simulink model "ControlRobot"  (R2018a)
settings: Solver=FixedStepAuto  StartTime=0.0  StopTime=3  FixedStep=T  RelTol=1e-3
values from neighbouring files (symbols this model uses):
  Bv = 0.055    [F.m]    (also in FNew.m = 0.038709; Project.m = 0.55; ProjectEdit.m = 0.55; SimulationWorkspace.m = 0.038709)
  Bvc = 0.038709    [SimulationWorkspace.m]
  Bw = 0.015    [F.m]    (also in FNew.m = 0.0008517; Project.m; ProjectEdit.m; SimulationWorkspace.m = 0.0008517)
  Bwc = 0.0008517    [SimulationWorkspace.m]
  Cv = 0.2    [F.m]    (also in FNew.m = 0.019178; Project.m = 2; ProjectEdit.m = 2; SimulationWorkspace.m = 0.019178)
  Cvc = 0.019178    [SimulationWorkspace.m]
  Cw = 0.14    [F.m]    (also in FNew.m = 0.099875; Project.m; ProjectEdit.m; SimulationWorkspace.m = 0.099875)
  Cwc = 0.099875    [SimulationWorkspace.m]
  eta1 = 1    [SimulationWorkspace.m]
  eta2 = 1    [SimulationWorkspace.m]
  eta3 = 0.1    [SimulationWorkspace.m]
  g = 9.81    [F.m]    (also in FNew.m; ForwardDynamicModel.m; Project.m; ProjectEdit.m)
  j = i + 1    [Fusion.m]
  J = 0.015    [F.m]    (also in FNew.m = 0.002; Jacobian.m = 0.5*[-S, -C, S, C; Project.m; ProjectEdit.m)
  Jc = 0.45923    [SimulationWorkspace.m]
  K1 = 2.5    [SimulationWorkspace.m]
  K2 = 2.5    [SimulationWorkspace.m]
  K3 = 20    [SimulationWorkspace.m]
  L = 0.1    [F.m]    (also in FNew.m = 0.15; H.m = 0.15; Project.m; ProjectEdit.m)
  lambda1 = 2.75    [SimulationWorkspace.m]
  lambda2 = 2.75    [SimulationWorkspace.m]
  lambda3 = 10    [SimulationWorkspace.m]
  M = 6    [F.m]    (also in FNew.m = 9.1; Project.m; ProjectEdit.m; SimulationWorkspace.m = 9.1)
  Mc = 9.1    [SimulationWorkspace.m]
  mu_p = 0    [SimulationWorkspace.m]
  Q = zeros(4, N - 1)    [Project.m]    (also in ProjectEdit.m; SimulationWorkspace.m = diag([0.002, 0.002, 3e-03, 0.002, 0.002, 3e-03]))
  r = 0.05    [F.m]    (also in FNew.m; H.m; Project.m; ProjectEdit.m)
  RG = diag([5e-7, 5e-7, 5e-7])    [SimulationWorkspace.m]
  RH = diag([2.5e-5, 2.5e-5, 2.5e-5, 2.5e-5])    [SimulationWorkspace.m]
  T = [1/29.56, 1/29.43, 1/30, 1/29.43, 1/29.78, 1/29.75, 1/29.8, 1/29.3, 1/29.18, 1/29.74, 1/29.29, 1/29.3, 1/29.73, 1/29.14, 1/29.75]    [DataRead.m]    (also in Encoder.m = 0.02; F.m = u(5); FNew.m = u(5); Fusion.m = 0.01)
libraries: simulink x4, sharedTrackingLibrary x1, dspsrcs4 x1
settings Model: Creator=Ammar Issa  LastModifiedBy=Ammar Issa
settings SolverCC: AlgebraicLoopSolver=LineSearch

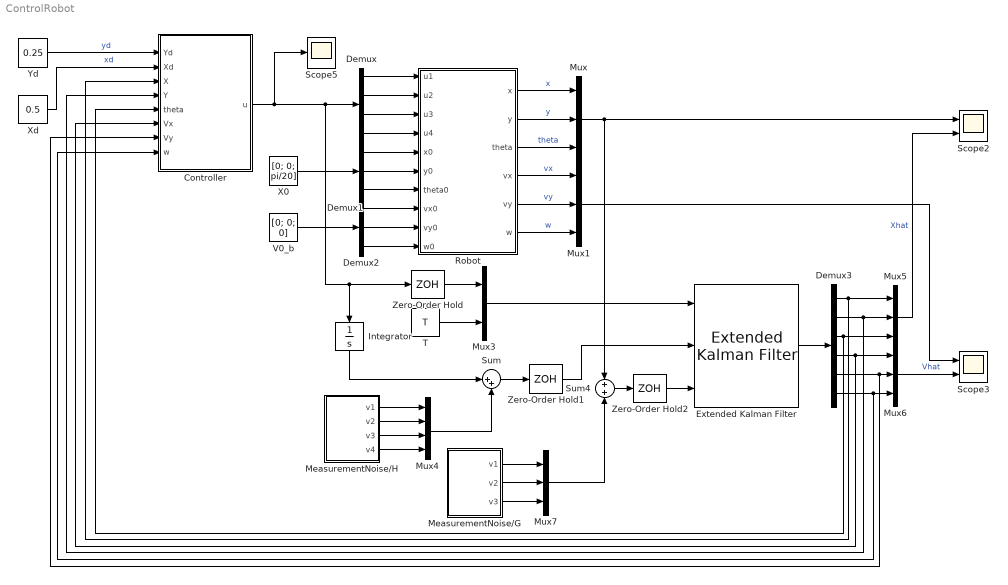
== system ControlRobot ==
  Controller : Subsystem
  Demux : Demux
  Demux1 : Demux  Outputs=3
  Demux2 : Demux  Outputs=3
  Demux3 : Demux  Outputs=6
  Extended Kalman Filter : sharedTrackingLibrary/Extended Kalman Filter  StateTransitionFcn=FNew  HasStateTransitionJacobianFcn=off  HasAdditiveProcessNoise=Additive  ProcessNoise=Q  HasTimeVaryingProcessNoise=off  HasStateTransitionFcnExtraArgument=1  InitialState=[0; 0; pi/20; 0; 0; 0]  InitialStateCovariance=diag([0,0,0,1e-6,1e-6,0])  MeasurementFcn1=H  HasMeasurementJacobianFcn1=off  HasMeasurementEnablePort1=off  HasAdditiveMeasurementNoise1=Additive  MeasurementNoise1=RH  HasTimeVaryingMeasurementNoise1=off  HasMeasurementFcnExtraArgument1=0  MeasurementFcn2=G  HasMeasurementJacobianFcn2=off  HasMeasurementEnablePort2=off  HasAdditiveMeasurementNoise2=Additive  MeasurementNoise2=RG  HasTimeVaryingMeasurementNoise2=off  HasMeasurementFcnExtraArgument2=0  MeasurementFcn3=myMeasurementFcn  HasMeasurementJacobianFcn3=off  HasMeasurementEnablePort3=off  HasAdditiveMeasurementNoise3=Additive  MeasurementNoise3=1  HasTimeVaryingMeasurementNoise3=off  HasMeasurementFcnExtraArgument3=0  MeasurementFcn4=myMeasurementFcn  HasMeasurementJacobianFcn4=off  HasMeasurementEnablePort4=off  HasAdditiveMeasurementNoise4=Additive  MeasurementNoise4=1  HasTimeVaryingMeasurementNoise4=off  HasMeasurementFcnExtraArgument4=0  MeasurementFcn5=myMeasurementFcn  HasMeasurementJacobianFcn5=off  HasMeasurementEnablePort5=off  HasAdditiveMeasurementNoise5=Additive  MeasurementNoise5=1  HasTimeVaryingMeasurementNoise5=off  HasMeasurementFcnExtraArgument5=0  EnableMultirate=on  StateTransitionFcnSampleTime=T  MeasurementFcn1SampleTime=T  MeasurementFcn2SampleTime=T  MeasurementFcn3SampleTime=1  MeasurementFcn4SampleTime=1  MeasurementFcn5SampleTime=1  UseCurrentEstimator=on  OutputStateCovariance=off  DataType=double  SampleTime=T  NumberOfMeasurements=2
      settings: SourceProductName=Control System Toolbox  SourceProductBaseCode=CT
  Integrator : Integrator
  MeasurementNoise/G : Subsystem
  MeasurementNoise/H : Subsystem
  Mux{,1,5..7} (5 alike) : Mux  Inputs=3
  Mux3 : Mux  Inputs=2
  Mux4 : Mux
  Robot : Subsystem
  Scope2 : Scope  NumInputPorts=2
  Scope3 : Scope  NumInputPorts=2
  Scope5 : Scope
  Sum : Sum  Inputs=|++
  Sum4 : Sum
  T : Constant  Value=T
  V0_b : Constant  Value=[0; 0; 0]
  X0 : Constant  Value=[0; 0; pi/20]
  Xd : Constant  Value=0.5
  Yd : Constant  Value=0.25
  Zero-Order Hold : ZeroOrderHold  SampleTime=T
  Zero-Order Hold1 : ZeroOrderHold  SampleTime=T
  Zero-Order Hold2 : ZeroOrderHold  SampleTime=T
  wires:
  Demux1/2 -> Robot/6(y0)
  Sum/1 -> Zero-Order Hold1/1
  Mux5/1 -> Scope2/2  "Xhat"
  T/1 -> Mux3/2
  MeasurementNoise/G/1(v1) -> Mux7/1
  MeasurementNoise/H/1(v1) -> Mux4/1
  Demux3/4 -> Controller/6(Vx), Mux6/1
  MeasurementNoise/H/3(v3) -> Mux4/3
  Mux6/1 -> Scope3/2  "Vhat"
  Mux7/1 -> Sum4/2
  Demux3/3 -> Controller/5(theta), Mux5/3
  Sum4/1 -> Zero-Order Hold2/1
  Demux2/2 -> Robot/9(vy0)
  Zero-Order Hold2/1 -> Extended Kalman Filter/3
  Zero-Order Hold1/1 -> Extended Kalman Filter/2
  Mux/1 -> Scope2/1, Sum4/1
  Zero-Order Hold/1 -> Mux3/1
  Extended Kalman Filter/1 -> Demux3/1
  Demux1/1 -> Robot/5(x0)
  Demux2/3 -> Robot/10(w0)
  Demux/2 -> Robot/2(u2)
  Demux/3 -> Robot/3(u3)
  Robot/4(vx) -> Mux1/1  "vx"
  MeasurementNoise/H/2(v2) -> Mux4/2
  Robot/3(theta) -> Mux/3  "theta"
  MeasurementNoise/H/4(v4) -> Mux4/4
  Robot/1(x) -> Mux/1  "x"
  Demux3/1 -> Controller/3(X), Mux5/1
  V0_b/1 -> Demux2/1
  Mux4/1 -> Sum/2
  Demux2/1 -> Robot/8(vx0)
  X0/1 -> Demux1/1
  MeasurementNoise/G/3(v3) -> Mux7/3
  Demux/1 -> Robot/1(u1)
  Demux3/6 -> Mux6/3, Controller/8(w)
  MeasurementNoise/G/2(v2) -> Mux7/2
  Demux1/3 -> Robot/7(theta0)
  Robot/6(w) -> Mux1/3  "w"
  Mux3/1 -> Extended Kalman Filter/1
  Demux/4 -> Robot/4(u4)
  Mux1/1 -> Scope3/1
  Demux3/5 -> Mux6/2, Controller/7(Vy)
  Robot/2(y) -> Mux/2  "y"
  Demux3/2 -> Controller/4(Y), Mux5/2
  Integrator/1 -> Sum/1
  Robot/5(vy) -> Mux1/2  "vy"
  Controller/1(u) -> Scope5/1, Integrator/1, Zero-Order Hold/1, Demux/1
  Yd/1 -> Controller/1(Yd)  "yd"
  Xd/1 -> Controller/2(Xd)  "xd"

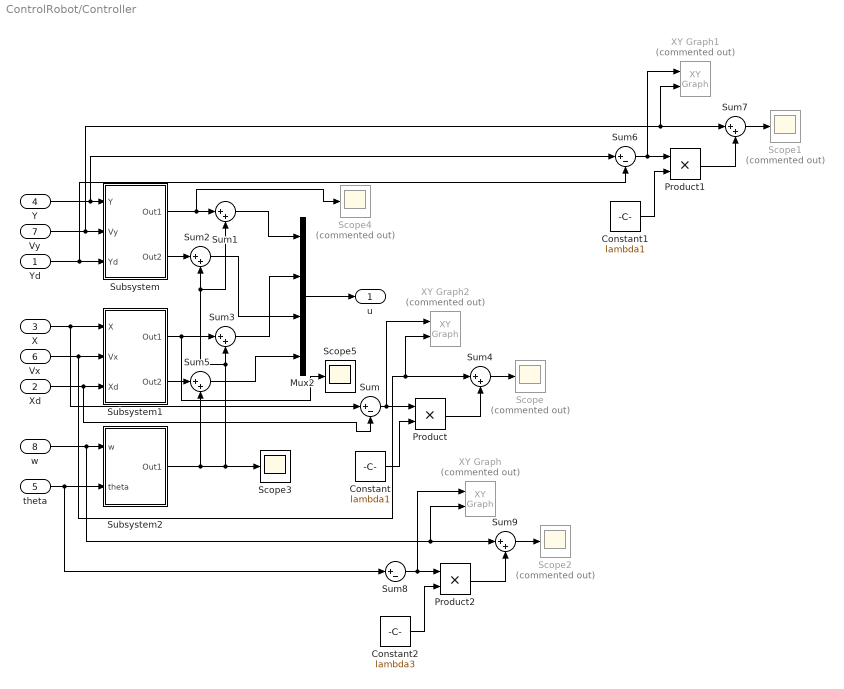
== system ControlRobot/Controller ==
  Yd : Inport
  Xd : Inport  Port=2
  X : Inport  Port=3
  Y : Inport  Port=4
  theta : Inport  Port=5
  Vx : Inport  Port=6
  Vy : Inport  Port=7
  w : Inport  Port=8
  Constant : Constant  Value=lambda1
  Constant1 : Constant  Value=lambda1
  Constant2 : Constant  Value=lambda3
  Mux2 : Mux
  Product : Product
  Product1 : Product
  Product2 : Product
  Scope{,1..2,4} (4 alike) : Scope  Commented=on
  Scope3 : Scope
  Scope5 : Scope
  Subsystem : Subsystem
  Subsystem1 : Subsystem
  Subsystem2 : Subsystem
  Sum : Sum  Inputs=|+-
  Sum{1..5,7,9} (7 alike) : Sum  Inputs=|++
  Sum6 : Sum  Inputs=|+-
  Sum8 : Sum  Inputs=|+-
  XY Graph : simulink/Sinks/XY Graph  Commented=on  xmin=-0.1  xmax=0.2  ymin=-0.05  ymax=0.05  st=-1
  XY Graph1 : simulink/Sinks/XY Graph  Commented=on  xmin=-0.6  xmax=0.1  ymin=-0.1  ymax=1.5  st=-1
  XY Graph2 : simulink/Sinks/XY Graph  Commented=on  xmin=-0.6  xmax=0.1  ymin=-0.1  ymax=1.5  st=-1
  u : Outport
  wires:
  Sum2/1 -> Mux2/3
  Subsystem2/1(Out1) -> Scope3/1, Sum1/2, Sum2/2, Sum3/2, Sum5/2
  Subsystem1/2(Out2) -> Sum5/1
  Subsystem1/1(Out1) -> Scope5/1, Sum3/1
  Subsystem/2(Out2) -> Sum2/1
  Subsystem/1(Out1) -> Scope4/1, Sum1/1
  Sum3/1 -> Mux2/2
  Sum5/1 -> Mux2/4
  Sum1/1 -> Mux2/1
  Xd/1 -> Sum/2, Subsystem1/3(Xd)
  Mux2/1 -> u/1
  Vx/1 -> XY Graph2/2, Sum4/1, Subsystem1/2(Vx)
  X/1 -> Sum/1, Subsystem1/1(X)
  Sum/1 -> XY Graph2/1, Product/1
  Constant/1 -> Product/2
  Product/1 -> Sum4/2
  Sum4/1 -> Scope/1
  Sum7/1 -> Scope1/1
  Product1/1 -> Sum7/2
  Constant1/1 -> Product1/2
  Sum6/1 -> Product1/1, XY Graph1/1
  Y/1 -> Sum6/1, Subsystem/1(Y)
  Vy/1 -> Sum7/1, XY Graph1/2, Subsystem/2(Vy)
  Yd/1 -> Sum6/2, Subsystem/3(Yd)
  Sum9/1 -> Scope2/1
  Product2/1 -> Sum9/2
  Constant2/1 -> Product2/2
  Sum8/1 -> XY Graph/1, Product2/1
  theta/1 -> Sum8/1, Subsystem2/2(theta)
  w/1 -> XY Graph/2, Sum9/1, Subsystem2/1(w)

== system ControlRobot/MeasurementNoise//G ==
  vw1 : RandomNumber  Variance=RG(1, 1)  Seed=4  SampleTime=0
  vw2 : RandomNumber  Variance=RG(2, 2)  Seed=5  SampleTime=0
  vw3 : RandomNumber  Variance=RG(3, 3)  Seed=6  SampleTime=0
  v1 : Outport
  v2 : Outport  Port=2
  v3 : Outport  Port=3
  wires:
  vw1/1 -> v1/1
  vw2/1 -> v2/1
  vw3/1 -> v3/1

== system ControlRobot/MeasurementNoise//H ==
  vw1 : RandomNumber  Variance=RH(1, 1)  SampleTime=0
  vw2 : RandomNumber  Variance=RH(2, 2)  Seed=1  SampleTime=0
  vw3 : RandomNumber  Variance=RH(3, 3)  Seed=2  SampleTime=0
  vw4 : RandomNumber  Variance=RH(4, 4)  Seed=3  SampleTime=0
  v1 : Outport
  v2 : Outport  Port=2
  v3 : Outport  Port=3
  v4 : Outport  Port=4
  wires:
  vw3/1 -> v3/1
  vw4/1 -> v4/1
  vw2/1 -> v2/1
  vw1/1 -> v1/1

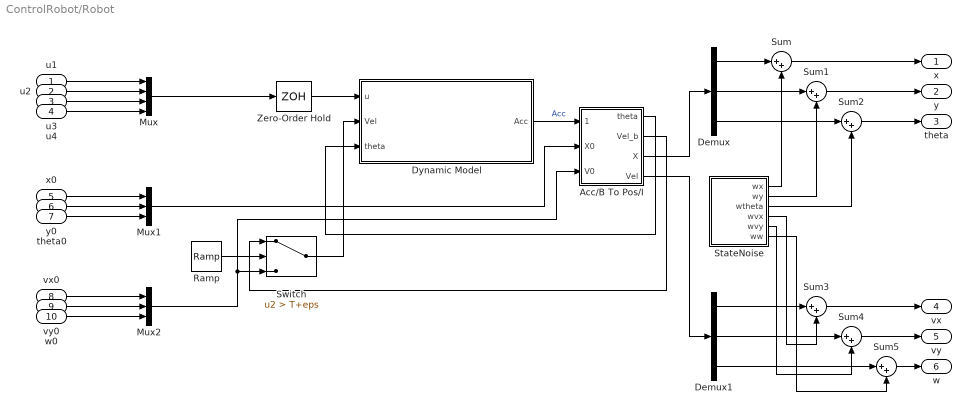
== system ControlRobot/Robot ==
  u1 : Inport
  u2 : Inport  Port=2
  u3 : Inport  Port=3
  u4 : Inport  Port=4
  x0 : Inport  Port=5
  y0 : Inport  Port=6
  theta0 : Inport  Port=7
  vx0 : Inport  Port=8
  vy0 : Inport  Port=9
  w0 : Inport  Port=10
  Acc/B To Pos/I : Subsystem
  Demux : Demux  Outputs=3
  Demux1 : Demux  Outputs=3
  Dynamic Model : Subsystem
  Mux : Mux
  Mux1 : Mux  Inputs=3
  Mux2 : Mux  Inputs=3
  Ramp : simulink/Sources/Ramp  slope=1  start=0  InitialOutput=0
  StateNoise : Subsystem
  Sum{,1..5} (6 alike) : Sum  Inputs=|++
  Switch : Switch  Criteria=u2 > Threshold  Threshold=T+eps
  Zero-Order Hold : ZeroOrderHold  SampleTime=T
  x : Outport
  y : Outport  Port=2
  theta : Outport  Port=3
  vx : Outport  Port=4
  vy : Outport  Port=5
  w : Outport  Port=6
  wires:
  Dynamic Model/1(Acc) -> Acc/B To Pos/I/1(Acc_b)  "Acc"
  Switch/1 -> Dynamic Model/2(Vel)
  Acc/B To Pos/I/1(theta) -> Dynamic Model/3(theta)
  Acc/B To Pos/I/3(X) -> Demux/1
  Mux2/1 -> Acc/B To Pos/I/3(V0), Switch/3
  vx0/1 -> Mux2/1
  Mux1/1 -> Acc/B To Pos/I/2(X0)
  Ramp/1 -> Switch/2
  Acc/B To Pos/I/2(Vel_b) -> Switch/1
  Acc/B To Pos/I/4(Vel) -> Demux1/1
  Mux/1 -> Zero-Order Hold/1
  vy0/1 -> Mux2/2
  u4/1 -> Mux/4
  u3/1 -> Mux/3
  w0/1 -> Mux2/3
  y0/1 -> Mux1/2
  x0/1 -> Mux1/1
  theta0/1 -> Mux1/3
  u2/1 -> Mux/2
  u1/1 -> Mux/1
  Demux/1 -> Sum/1
  Demux/2 -> Sum1/1
  Demux/3 -> Sum2/1
  Demux1/3 -> Sum5/1
  Demux1/2 -> Sum4/1
  Demux1/1 -> Sum3/1
  StateNoise/1(wx) -> Sum/2
  StateNoise/2(wy) -> Sum1/2
  StateNoise/3(wtheta) -> Sum2/2
  StateNoise/4(wvx) -> Sum3/2
  StateNoise/5(wvy) -> Sum4/2
  StateNoise/6(ww) -> Sum5/2
  Sum5/1 -> w/1
  Sum4/1 -> vy/1
  Sum3/1 -> vx/1
  Sum2/1 -> theta/1
  Sum1/1 -> y/1
  Sum/1 -> x/1
  Zero-Order Hold/1 -> Dynamic Model/1(u)

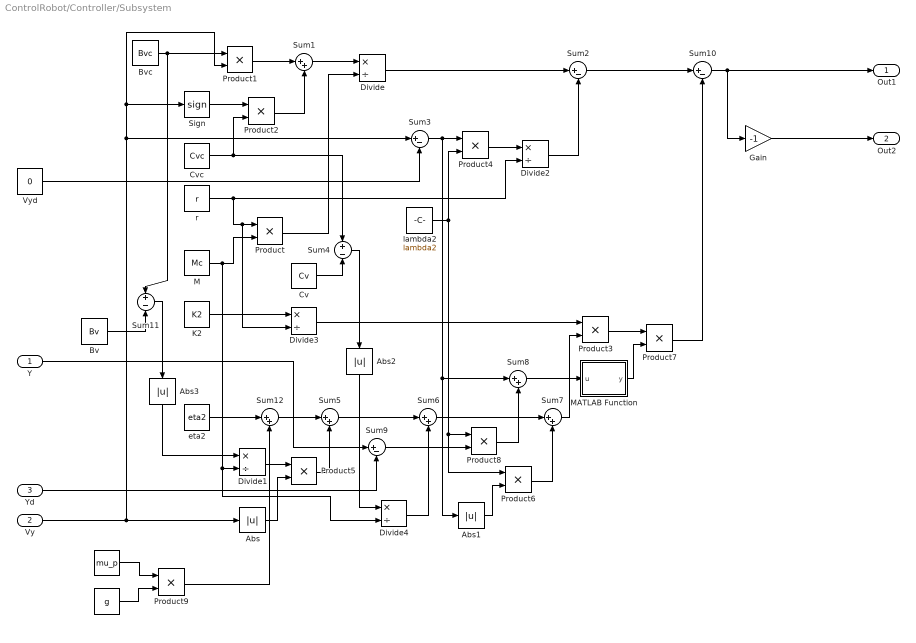
== system ControlRobot/Controller/Subsystem ==
  Y : Inport
  Vy : Inport  Port=2
  Yd : Inport  Port=3
  " " : Constant  Value=mu_p
  "  " : Constant  Value=g
  Abs{,1..3} (4 alike) : Abs
  Bv : Constant  Value=Bv
  Bvc : Constant  Value=Bvc
  Cv : Constant  Value=Cv
  Cvc : Constant  Value=Cvc
  Divide{,1..4} (5 alike) : Product  Inputs=*/
  Gain : Gain  Gain=-1
  K2 : Constant  Value=K2
  M : Constant  Value=Mc
  MATLAB Function : MATLAB Function  TreatAsAtomicUnit=on
  Product{,1..9} (10 alike) : Product
  Sign : Signum
  Sum{1,5..8,12} (6 alike) : Sum  Inputs=|++
  Sum{2..3,9..10} (4 alike) : Sum  Inputs=|+-
  Sum11 : Sum  Inputs=+-
  Sum4 : Sum  Inputs=+-
  Vyd : Constant  Value=0
  eta2 : Constant  Value=eta2
  lambda2 : Constant  Value=lambda2
  r : Constant  Value=r
  Out1 : Outport
  Out2 : Outport  Port=2
  wires:
  Divide4/1 -> Sum6/2
  Product4/1 -> Divide2/1
  Bvc/1 -> Sum11/1, Product1/1
  Divide/1 -> Sum2/1
  Sum1/1 -> Divide/1
  Vy/1 -> Sign/1, Product1/2, Sum3/1, Abs/1
  Sum5/1 -> Sum6/1
  Product3/1 -> Product7/1
  Abs1/1 -> Product6/2
  Product8/1 -> Sum8/2
  Sum9/1 -> Product8/2
  Sum3/1 -> Sum8/1, Abs1/1, Product4/1
  Abs/1 -> Product5/2
  Sum7/1 -> Product3/2
  lambda2/1 -> Product8/1, Product6/1, Product4/2
  Product7/1 -> Sum10/2
  Y/1 -> Sum9/1
  Product1/1 -> Sum1/1
  MATLAB Function/1(y) -> Product7/2
  Sum6/1 -> Sum7/1
  Sum2/1 -> Sum10/1
  M/1 -> Divide1/2, Divide4/2, Product/2
  Product6/1 -> Sum7/2
  Sign/1 -> Product2/1
  Sum10/1 -> Out1/1, Gain/1
  r/1 -> Divide2/2, Divide3/2, Product/1
  Product2/1 -> Sum1/2
  Divide1/1 -> Product5/1
  Product5/1 -> Sum5/2
  Product/1 -> Divide/2
  Divide2/1 -> Sum2/2
  Cvc/1 -> Sum4/1, Product2/2
  K2/1 -> Divide3/1
  Divide3/1 -> Product3/1
  Yd/1 -> Sum9/2
  Gain/1 -> Out2/1
  Vyd/1 -> Sum3/2
  Sum8/1 -> MATLAB Function/1(u)
  Cv/1 -> Sum4/2
  Sum4/1 -> Abs2/1
  Abs2/1 -> Divide4/1
  Bv/1 -> Sum11/2
  Sum11/1 -> Abs3/1
  Abs3/1 -> Divide1/1
  eta2/1 -> Sum12/1
  Sum12/1 -> Sum5/1
  " "/1 -> Product9/1
  "  "/1 -> Product9/2
  Product9/1 -> Sum12/2

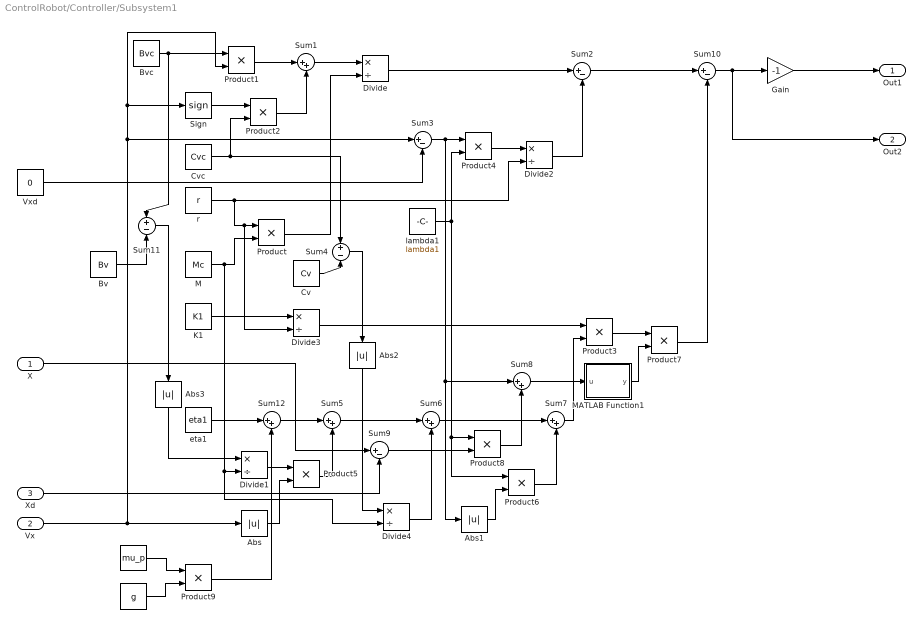
== system ControlRobot/Controller/Subsystem1 ==
  X : Inport
  Vx : Inport  Port=2
  Xd : Inport  Port=3
  " " : Constant  Value=mu_p
  "  " : Constant  Value=g
  Abs{,1..3} (4 alike) : Abs
  Bv : Constant  Value=Bv
  Bvc : Constant  Value=Bvc
  Cv : Constant  Value=Cv
  Cvc : Constant  Value=Cvc
  Divide{,1..4} (5 alike) : Product  Inputs=*/
  Gain : Gain  Gain=-1
  K1 : Constant  Value=K1
  M : Constant  Value=Mc
  MATLAB Function1 : MATLAB Function  TreatAsAtomicUnit=on
  Product{,1..9} (10 alike) : Product
  Sign : Signum
  Sum{1,5..8,12} (6 alike) : Sum  Inputs=|++
  Sum{2..3,9..10} (4 alike) : Sum  Inputs=|+-
  Sum11 : Sum  Inputs=+-
  Sum4 : Sum  Inputs=+-
  Vxd : Constant  Value=0
  eta1 : Constant  Value=eta1
  lambda1 : Constant  Value=lambda1
  r : Constant  Value=r
  Out1 : Outport
  Out2 : Outport  Port=2
  wires:
  Vxd/1 -> Sum3/2
  Sum10/1 -> Out2/1, Gain/1
  Xd/1 -> Sum9/2
  Divide3/1 -> Product3/1
  K1/1 -> Divide3/1
  Cvc/1 -> Sum4/1, Product2/2
  Divide2/1 -> Sum2/2
  Product/1 -> Divide/2
  Product5/1 -> Sum5/2
  Divide1/1 -> Product5/1
  Product2/1 -> Sum1/2
  r/1 -> Product/1, Divide3/2, Divide2/2
  Sum8/1 -> MATLAB Function1/1(u)
  Product6/1 -> Sum7/2
  M/1 -> Product/2, Divide4/2, Divide1/2
  Sum2/1 -> Sum10/1
  Sum6/1 -> Sum7/1
  Product1/1 -> Sum1/1
  X/1 -> Sum9/1
  Product7/1 -> Sum10/2
  lambda1/1 -> Product4/2, Product6/1, Product8/1
  Sum7/1 -> Product3/2
  Abs/1 -> Product5/2
  Sum3/1 -> Product4/1, Abs1/1, Sum8/1
  Sum9/1 -> Product8/2
  Product8/1 -> Sum8/2
  Abs1/1 -> Product6/2
  Product3/1 -> Product7/1
  Sum5/1 -> Sum6/1
  Vx/1 -> Abs/1, Sum3/1, Sign/1, Product1/2
  Sum1/1 -> Divide/1
  Divide/1 -> Sum2/1
  Bvc/1 -> Sum11/1, Product1/1
  Product4/1 -> Divide2/1
  Divide4/1 -> Sum6/2
  Gain/1 -> Out1/1
  MATLAB Function1/1(y) -> Product7/2
  Sign/1 -> Product2/1
  Cv/1 -> Sum4/2
  Sum4/1 -> Abs2/1
  Abs2/1 -> Divide4/1
  Bv/1 -> Sum11/2
  Sum11/1 -> Abs3/1
  Abs3/1 -> Divide1/1
  "  "/1 -> Product9/2
  Product9/1 -> Sum12/2
  " "/1 -> Product9/1
  eta1/1 -> Sum12/1
  Sum12/1 -> Sum5/1

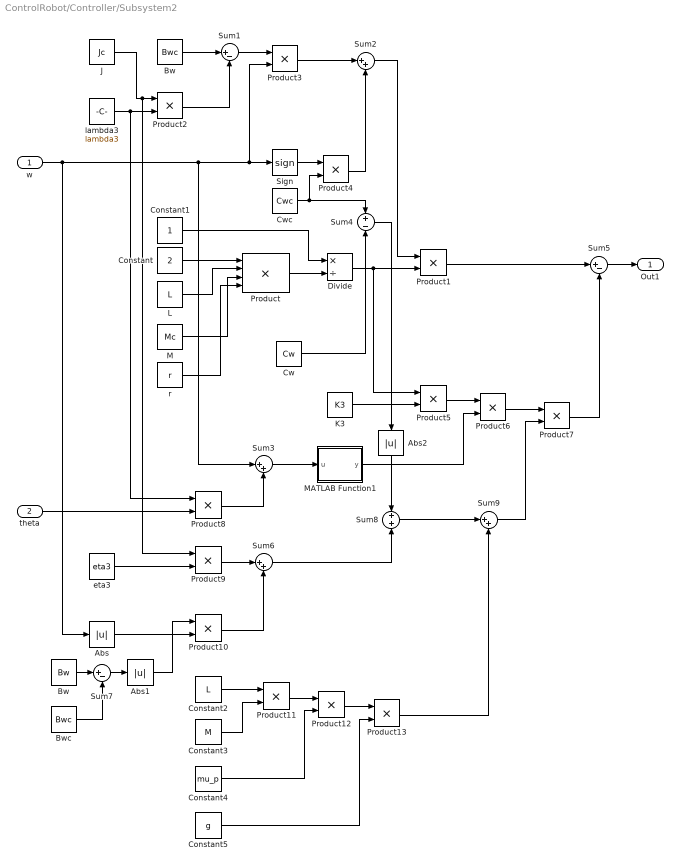
== system ControlRobot/Controller/Subsystem2 ==
  w : Inport
  theta : Inport  Port=2
  Abs : Abs
  Abs1 : Abs
  Abs2 : Abs
  Bw : Constant  Value=Bwc
  "Bw " : Constant  Value=Bw
  Bwc : Constant  Value=Bwc
  Constant : Constant  Value=2
  Constant1 : Constant
  Constant2 : Constant  Value=L
  Constant3 : Constant  Value=M
  Constant4 : Constant  Value=mu_p
  Constant5 : Constant  Value=g
  Cw : Constant  Value=Cw
  Cwc : Constant  Value=Cwc
  Divide : Product  Inputs=*/
  J : Constant  Value=Jc
  K3 : Constant  Value=K3
  L : Constant  Value=L
  M : Constant  Value=Mc
  MATLAB Function1 : MATLAB Function  TreatAsAtomicUnit=on
  Product : Product  Inputs=4
  Product{1..13} (13 alike) : Product
  Sign : Signum
  Sum1 : Sum  Inputs=|+-
  Sum{2..3,6,9} (4 alike) : Sum  Inputs=|++
  Sum4 : Sum  Inputs=+-
  Sum5 : Sum  Inputs=|+-
  Sum7 : Sum  Inputs=|+-
  Sum8 : Sum
  eta3 : Constant  Value=eta3
  lambda3 : Constant  Value=lambda3
  r : Constant  Value=r
  Out1 : Outport
  wires:
  theta/1 -> Product8/2
  w/1 -> Abs/1, Sum3/1, Sign/1, Product3/2
  Bw/1 -> Sum1/1
  K3/1 -> Product5/2
  Sum7/1 -> Abs1/1
  J/1 -> Product9/1, Product2/1
  Product5/1 -> Product6/1
  Product1/1 -> Sum5/1
  Product2/1 -> Sum1/2
  Abs/1 -> Product10/2
  Product/1 -> Divide/2
  Product6/1 -> Product7/1
  L/1 -> Product/2
  Sum6/1 -> Sum8/2
  Constant1/1 -> Divide/1
  Product7/1 -> Sum5/2
  Product4/1 -> Sum2/2
  Product8/1 -> Sum3/2
  Sign/1 -> Product4/1
  Cwc/1 -> Sum4/1, Product4/2
  Sum5/1 -> Out1/1
  Divide/1 -> Product5/1, Product1/2
  Product3/1 -> Sum2/1
  lambda3/1 -> Product8/1, Product2/2
  Sum2/1 -> Product1/1
  r/1 -> Product/4
  Constant/1 -> Product/1
  M/1 -> Product/3
  eta3/1 -> Product9/2
  Product9/1 -> Sum6/1
  Bwc/1 -> Sum7/2
  Product10/1 -> Sum6/2
  Sum1/1 -> Product3/1
  "Bw "/1 -> Sum7/1
  Abs1/1 -> Product10/1
  Cw/1 -> Sum4/2
  Sum4/1 -> Abs2/1
  Abs2/1 -> Sum8/1
  Sum8/1 -> Sum9/1
  Sum9/1 -> Product7/2
  Constant2/1 -> Product11/1
  Constant3/1 -> Product11/2
  Product11/1 -> Product12/1
  Constant4/1 -> Product12/2
  Product12/1 -> Product13/1
  Constant5/1 -> Product13/2
  Product13/1 -> Sum9/2
  Sum3/1 -> MATLAB Function1/1(u)
  MATLAB Function1/1(y) -> Product6/2

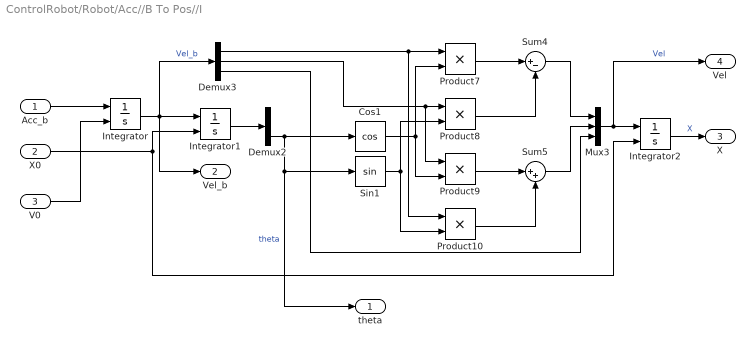
== system ControlRobot/Robot/Acc//B To Pos//I ==
  Acc_b : Inport
  X0 : Inport  Port=2
  V0 : Inport  Port=3
  Cos1 : Trigonometry  Operator=cos
  Demux2 : Demux  Outputs=3
  Demux3 : Demux  Outputs=3
  Integrator : Integrator  InitialConditionSource=external
  Integrator1 : Integrator  InitialConditionSource=external
  Integrator2 : Integrator  InitialConditionSource=external
  Mux3 : Mux  Inputs=3
  Product{7..10} (4 alike) : Product
  Sin1 : Trigonometry
  Sum4 : Sum  Inputs=|+-
  Sum5 : Sum  Inputs=|++
  theta : Outport
  Vel_b : Outport  Port=2
  X : Outport  Port=3
  Vel : Outport  Port=4
  wires:
  Demux3/2 -> Product9/1, Product8/1
  Integrator/1 -> Integrator1/1, Vel_b/1, Demux3/1  "Vel_b"
  Demux3/3 -> Mux3/3
  Demux2/3 -> Cos1/1, theta/1, Sin1/1  "theta"
  Integrator1/1 -> Demux2/1
  Cos1/1 -> Product9/2, Product7/2
  Demux3/1 -> Product10/1, Product7/1
  Sum5/1 -> Mux3/2
  Product8/1 -> Sum4/2
  Integrator2/1 -> X/1  "X"
  Product7/1 -> Sum4/1
  Sin1/1 -> Product10/2, Product8/2
  Sum4/1 -> Mux3/1
  Product10/1 -> Sum5/2
  Product9/1 -> Sum5/1
  Mux3/1 -> Integrator2/1, Vel/1  "Vel"
  Acc_b/1 -> Integrator/1
  V0/1 -> Integrator/2
  X0/1 -> Integrator2/2, Integrator1/2

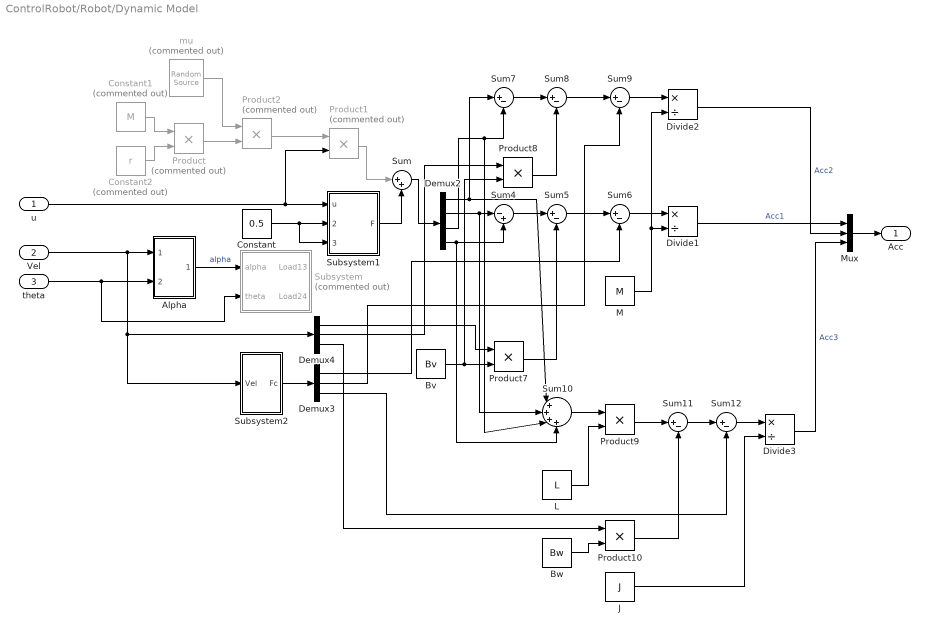
== system ControlRobot/Robot/Dynamic Model ==
  u : Inport
  Vel : Inport  Port=2
  theta : Inport  Port=3
  Alpha : Subsystem
  Bv : Constant  Value=Bv
  Bw : Constant  Value=Bw
  Constant : Constant  Value=0.5
  Constant1 : Constant  Commented=on  Value=M
  Constant2 : Constant  Commented=on  Value=r
  Demux2 : Demux
  Demux3 : Demux  Outputs=3
  Demux4 : Demux  Outputs=3
  Divide1 : Product  Inputs=*/
  Divide2 : Product  Inputs=*/
  Divide3 : Product  Inputs=*/
  J : Constant  Value=J
  L : Constant  Value=L
  M : Constant  Value=M
  Mux : Mux  Inputs=3
  Product : Product  Commented=on
  Product1 : Product  Commented=on
  Product{7..10} (4 alike) : Product
  Product2 : Product  Commented=on
  Subsystem : Subsystem  Commented=on
  Subsystem1 : Subsystem
  Subsystem2 : Subsystem
  Sum : Sum  Inputs=|++
  Sum10 : Sum  Inputs=|++++
  Sum{5..9,11..12} (7 alike) : Sum  Inputs=|+-
  Sum4 : Sum  Inputs=|-+
  mu : dspsrcs4/Random Source  Commented=on  SrcType=Uniform  NormMethod=Ziggurat  CltLength=12  MinVal=-0.2  MaxVal=0.2  MeanVal=0  VarVal=1  RepMode=Not repeatable  rawSeed=1  IsInherit=off  SampMode=Continuous  SampTime=T  SampFrame=1  DataType=Double  OutComplex=Real  OutputFrames=off
  Acc : Outport
  wires:
  Sum7/1 -> Sum8/1
  Vel/1 -> Demux4/1, Subsystem2/1(Vel), Alpha/1(Vel)
  Sum8/1 -> Sum9/1
  theta/1 -> Alpha/2(theta), Subsystem/2(theta)
  u/1 -> Product1/2, Subsystem1/1(u)
  Product7/1 -> Sum5/2
  Sum9/1 -> Divide2/1
  Demux4/2 -> Product8/1
  J/1 -> Divide3/2
  Subsystem2/1(Fc) -> Demux3/1
  Alpha/1(alpha) -> Subsystem/1(alpha)  "alpha"
  Demux4/3 -> Product10/1
  Bv/1 -> Product7/2, Product8/2
  Demux3/1 -> Sum6/2
  Demux2/2 -> Sum10/2, Sum4/1
  Demux3/2 -> Sum9/2
  M/1 -> Divide1/2, Divide2/2
  Product9/1 -> Sum11/1
  Divide3/1 -> Mux/3  "Acc3"
  Sum6/1 -> Divide1/1
  Sum5/1 -> Sum6/1
  Demux2/3 -> Sum10/3, Sum7/2
  Sum10/1 -> Product9/1
  Product8/1 -> Sum8/2
  Demux2/1 -> Sum10/1, Sum7/1
  Demux4/1 -> Product7/1
  Sum12/1 -> Divide3/1
  Demux2/4 -> Sum4/2, Sum10/4
  Sum4/1 -> Sum5/1
  L/1 -> Product9/2
  Sum11/1 -> Sum12/1
  Demux3/3 -> Sum12/2
  Bw/1 -> Product10/2
  Product10/1 -> Sum11/2
  Divide1/1 -> Mux/1  "Acc1"
  Divide2/1 -> Mux/2  "Acc2"
  Mux/1 -> Acc/1
  Constant/1 -> Subsystem1/3(Load24), Subsystem1/2(Load13)
  Sum/1 -> Demux2/1
  Subsystem1/1(F) -> Sum/2
  Constant1/1 -> Product/1
  Constant2/1 -> Product/2
  Product1/1 -> Sum/1
  Product/1 -> Product2/2
  mu/1 -> Product2/1
  Product2/1 -> Product1/1

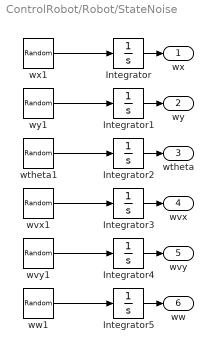
== system ControlRobot/Robot/StateNoise ==
  Integrator{,1..5} (6 alike) : Integrator
  wtheta1 : RandomNumber  Variance=Q(3, 3)  Seed=8  SampleTime=0
  wvx1 : RandomNumber  Variance=Q(4, 4)  Seed=9  SampleTime=0
  wvy1 : RandomNumber  Variance=Q(5, 5)  Seed=10  SampleTime=0
  ww1 : RandomNumber  Variance=Q(6, 6)  Seed=11  SampleTime=0
  wx1 : RandomNumber  Variance=Q(1, 1)  Seed=6  SampleTime=0
  wy1 : RandomNumber  Variance=Q(2, 2)  Seed=7  SampleTime=0
  wx : Outport
  wy : Outport  Port=2
  wtheta : Outport  Port=3
  wvx : Outport  Port=4
  wvy : Outport  Port=5
  ww : Outport  Port=6
  wires:
  Integrator2/1 -> wtheta/1
  Integrator3/1 -> wvx/1
  Integrator1/1 -> wy/1
  wx1/1 -> Integrator/1
  Integrator5/1 -> ww/1
  wvx1/1 -> Integrator3/1
  wtheta1/1 -> Integrator2/1
  wy1/1 -> Integrator1/1
  ww1/1 -> Integrator5/1
  wvy1/1 -> Integrator4/1
  Integrator/1 -> wx/1
  Integrator4/1 -> wvy/1

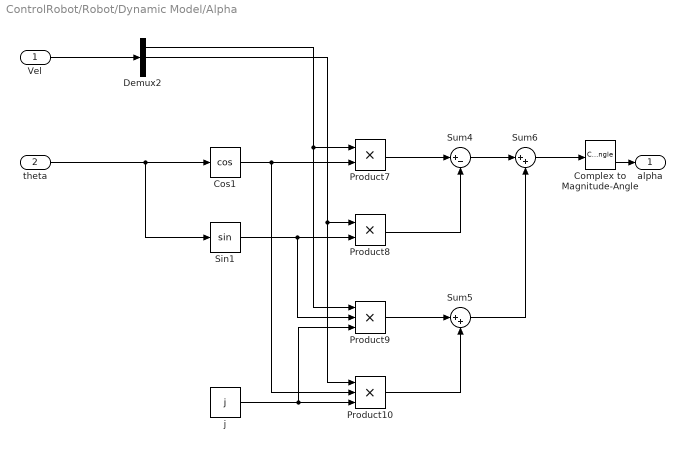
== system ControlRobot/Robot/Dynamic Model/Alpha ==
  Vel : Inport
  theta : Inport  Port=2
  Complex to Magnitude-Angle : ComplexToMagnitudeAngle
  Cos1 : Trigonometry  Operator=cos
  Demux2 : Demux  Outputs=3
  Product10 : Product  Inputs=3
  Product7 : Product
  Product8 : Product
  Product9 : Product  Inputs=3
  Sin1 : Trigonometry
  Sum4 : Sum  Inputs=|+-
  Sum5 : Sum  Inputs=|++
  Sum6 : Sum  Inputs=|++
  j : Constant  Value=j
  alpha : Outport
  wires:
  Product10/1 -> Sum5/2
  Demux2/1 -> Product9/1, Product7/1
  Sin1/1 -> Product9/2, Product8/2
  Product8/1 -> Sum4/2
  theta/1 -> Sin1/1, Cos1/1
  Cos1/1 -> Product10/2, Product7/2
  Sum4/1 -> Sum6/1
  Demux2/2 -> Product10/1, Product8/1
  Complex to Magnitude-Angle/2 -> alpha/1
  Sum6/1 -> Complex to Magnitude-Angle/1
  Product9/1 -> Sum5/1
  j/1 -> Product9/3, Product10/3
  Sum5/1 -> Sum6/2
  Product7/1 -> Sum4/1
  Vel/1 -> Demux2/1

== system ControlRobot/Robot/Dynamic Model/Subsystem ==
  alpha : Inport
  theta : Inport  Port=2
  Demux : Demux  Outputs=2
  MATLAB Function : MATLAB Function  TreatAsAtomicUnit=on
  Sum4 : Sum  Inputs=|+-
  Load13 : Outport
  Load24 : Outport  Port=2
  wires:
  alpha/1 -> Sum4/1
  Demux/1 -> Load13/1  "Load13"
  theta/1 -> Sum4/2
  Demux/2 -> Load24/1  "Load24"
  Sum4/1 -> MATLAB Function/1(beta)
  MATLAB Function/1(y) -> Demux/1

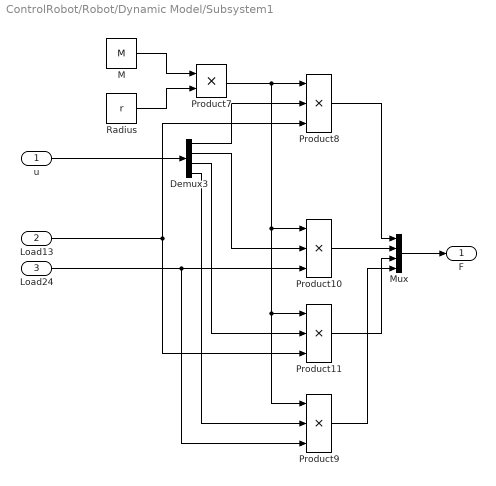
== system ControlRobot/Robot/Dynamic Model/Subsystem1 ==
  u : Inport
  Load13 : Inport  Port=2
  Load24 : Inport  Port=3
  Demux3 : Demux
  M : Constant  Value=M
  Mux : Mux
  Product{8..11} (4 alike) : Product  Inputs=3
  Product7 : Product
  Radius : Constant  Value=r
  F : Outport
  wires:
  Radius/1 -> Product7/2
  Load13/1 -> Product11/3, Product8/3
  Product7/1 -> Product9/1, Product11/1, Product10/1, Product8/1
  Product9/1 -> Mux/4
  Demux3/3 -> Product11/2
  M/1 -> Product7/1
  Demux3/1 -> Product8/2
  Demux3/2 -> Product10/2
  Demux3/4 -> Product9/2
  Product10/1 -> Mux/2
  Product11/1 -> Mux/3
  u/1 -> Demux3/1
  Load24/1 -> Product9/3, Product10/3
  Product8/1 -> Mux/1
  Mux/1 -> F/1

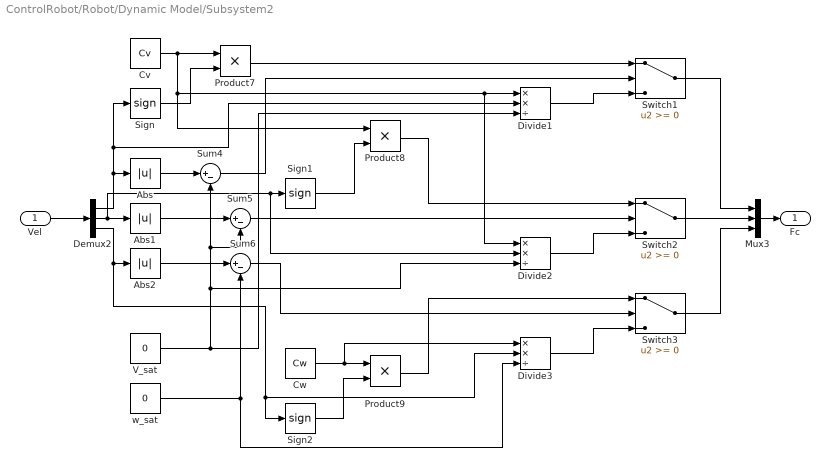
== system ControlRobot/Robot/Dynamic Model/Subsystem2 ==
  Vel : Inport
  Abs : Abs
  Abs1 : Abs
  Abs2 : Abs
  Cv : Constant  Value=Cv
  Cw : Constant  Value=Cw
  Demux2 : Demux  Outputs=3
  Divide1 : Product  Inputs=**/
  Divide2 : Product  Inputs=**/
  Divide3 : Product  Inputs=**/
  Mux3 : Mux  Inputs=3
  Product7 : Product
  Product8 : Product
  Product9 : Product
  Sign : Signum
  Sign1 : Signum
  Sign2 : Signum
  Sum4 : Sum  Inputs=|+-
  Sum5 : Sum  Inputs=|+-
  Sum6 : Sum  Inputs=|+-
  Switch1 : Switch
  Switch2 : Switch
  Switch3 : Switch
  V_sat : Constant  Value=0
  w_sat : Constant  Value=0
  Fc : Outport
  wires:
  Product8/1 -> Switch2/1
  Vel/1 -> Demux2/1
  Abs2/1 -> Sum6/1
  Cw/1 -> Divide3/1, Product9/1
  Demux2/3 -> Divide3/2, Sign2/1, Abs2/1
  Switch3/1 -> Mux3/3
  V_sat/1 -> Divide1/3, Divide2/3, Sum5/2, Sum4/2
  Cv/1 -> Product8/1, Divide2/1, Divide1/1, Product7/1
  Sign/1 -> Product7/2
  Demux2/2 -> Abs1/1, Divide2/2, Sign1/1
  Mux3/1 -> Fc/1
  Sign2/1 -> Product9/2
  Demux2/1 -> Divide1/2, Sign/1, Abs/1
  Sum5/1 -> Switch2/2
  w_sat/1 -> Divide3/3, Sum6/2
  Product9/1 -> Switch3/1
  Divide3/1 -> Switch3/3
  Divide2/1 -> Switch2/3
  Sum6/1 -> Switch3/2
  Abs/1 -> Sum4/1
  Divide1/1 -> Switch1/3
  Sum4/1 -> Switch1/2
  Switch1/1 -> Mux3/1
  Abs1/1 -> Sum5/1
  Sign1/1 -> Product8/2
  Switch2/1 -> Mux3/2
  Product7/1 -> Switch1/1

== matlab function ControlRobot/Controller/Subsystem/MATLAB Function ==
  data: u input; y output
function y = sat(u)
    u_sat = 0.04;
    y_sat = 1;
    if(u <= -u_sat)
        y = -y_sat;
    elseif(u >= u_sat)
        y = y_sat;
    else
        y = (y_sat/u_sat)*u;
    end
end

== matlab function ControlRobot/Robot/Dynamic Model/Subsystem/MATLAB Function ==
  data: beta input; y output
function y = fcn(beta)
    Load13 = 0;
    if(beta < 0)
        beta = beta + 2*pi;
    end
%     if((beta >= 0 && beta <= pi/2))
%         Load13 = beta/pi;
%     elseif(beta >= pi/2 && beta <= pi)
%         Load13 = 1 - beta/pi;
%     elseif(beta >= pi && beta <= 3*pi/2)
%         Load13 = -1 + beta/pi;
%     elseif(beta >= 3*pi/2 && beta <= 2*pi)
%         Load13 = -beta/pi + 2;
%     end
%     Load24 = 0.5 - Load13;
    Load24 = 0;
    if(beta >= 0 && beta <= pi/4)
        Load13 = 2*beta/pi;
    elseif(beta >= pi/4 && beta <= 3*pi/4)
        Load13 = 0.5;
    elseif(beta >= 3*pi/4 && beta <= pi)
        Load13 = 2 - 2*beta/pi;
    elseif(beta >= pi && beta <= pi + pi/4)
        Load13 = 2*(beta - pi)/pi;
    elseif(beta >= pi + pi/4 && beta <= pi + 3*pi/4)
        Load13 = 0.5;
    elseif(beta >= pi + 3*pi/4 && beta <= 2*pi)
        Load13 = 2 - 2*(beta - pi)/pi;
    end
    if(beta >= 0 && beta <= pi/4)
        Load24 = 0.5;
    elseif(beta >= pi/4 && beta <= pi/2)
        Load24 = -2*(beta - pi/4)/pi + 0.5;
    elseif(beta >= pi/2 && beta <= 3*pi/4)
        Load24 = 2*(beta - pi/2)/pi;
    elseif(beta >= 3*pi/4 && beta <= 3*pi/4 + pi/2)
        Load24 = 0.5;
    elseif(beta >= 3*pi/4 + pi/2 && beta <= 3*pi/4 + pi/2 + pi/4)
        Load24 = -2*(beta - pi/4 - pi)/pi + 0.5;
    elseif(beta >= 3*pi/4 + pi/2 + pi/4 && beta <= 3*pi/4 + pi/2 + 2*pi/4)
        Load24 = 2*(beta - 2*pi/4 - pi)/pi;
    elseif(beta >= 3*pi/4 + pi/2 + 2*pi/4 && beta <= 2*pi)
        Load24 = 0.5;
    end
    y = [Load13, Load24];
end

== matlab function ControlRobot/Controller/Subsystem2/MATLAB Function1 ==
  data: u input; y output
function y = sat(u)
    u_sat = 0.12;
    y_sat = 1;
    if(u <= -u_sat)
        y = -y_sat;
    elseif(u >= u_sat)
        y = y_sat;
    else
        y = (y_sat/u_sat)*u;
    end
end

== matlab function ControlRobot/Controller/Subsystem1/MATLAB Function1 ==
  data: u input; y output
function y = sat(u)
    u_sat = 0.04;
    y_sat = 1;
    if(u <= -u_sat)
        y = -y_sat;
    elseif(u >= u_sat)
        y = y_sat;
    else
        y = (y_sat/u_sat)*u;
    end
end
